simulink model "KD_cl_harness_forthao"  (R2015a)
settings: Solver=ode45  StartTime=0  StopTime=50  FixedStep=0.01  MaxStep=0.005  RelTol=1e-4  AbsTol=1e-4
InitFcn:
  | load KD_const_coeffs_0624
  | load pexhat_stuff
  | load expcon
  | load thr_ff_map
values from neighbouring files (symbols this model uses):
  c_0 = 0    [expcon.mat]
  c_1 = 1    [expcon.mat]
  c_100 = 100    [expcon.mat]
  c_1000 = 1000    [expcon.mat]
  c_10000 = 10000    [expcon.mat]
  c_1000inv = 0.0010000000475    [expcon.mat]    (also in pexhat_stuff.mat)
  c_100inv = 0.00999999977648    [expcon.mat]
  c_1_int = 1    [expcon.mat]
  c_1d2p4 = 0.416666656733    [expcon.mat]
  c_1p7 = 1.70000004768    [expcon.mat]
  c_4400inv = 0.000227272728807    [pexhat_stuff.mat]
  c_5500inv = 0.000181818177225    [expcon.mat]
  c_80 = 80    [expcon.mat]
  c_90 = 90    [expcon.mat]
  c_cal_phi = 7.6395999713e-06    [expcon.mat]
  c_compmap = [28125.0058594 29577.4082031 31350.1035156 33776.21875 37051.9296875 41026.2695312 45453.9960938 50160.3515625 55029.671875 59986.109375 64980.4296875 69980.4375 ... (320 elements, 20x16)]    [expcon.mat]
  c_ctok = 273.149993896    [expcon.mat]
  c_fflow_max = inf    [expcon.mat]
  c_fflow_min = 0    [expcon.mat]
  c_filt = 0.949999988079    [expcon.mat]
  c_flowdiv = 9.99999974738e-05    [expcon.mat]
  c_flowmin = 0    [expcon.mat]
  c_flowmult = 10000    [expcon.mat]
  c_inf = inf    [expcon.mat]
  c_km1d2k = 0.142857149243    [expcon.mat]
  c_mm3tokgpers = 2.77333338516e-08    [expcon.mat]
  c_n1 = -1    [expcon.mat]
  c_p00001 = 9.99999974738e-06    [expcon.mat]
  c_p01 = 0.00999999977648    [pexhat_stuff.mat]
  c_p016 = 0.01600000076    [expcon.mat]
  c_p1429 = 0.142900004983    [expcon.mat]
  c_p1e9 = 9.99999971718e-10    [expcon.mat]
  c_p4167 = 0.416700005531    [expcon.mat]    (also in pexhat_stuff.mat = 0.416666656733)
  c_p4d1p4 = 0.285714298487    [expcon.mat]
  c_p5401 = 0.540099978447    [expcon.mat]
  c_p9 = 0.899999976158    [expcon.mat]
  c_pincomp = 97.4216003418    [expcon.mat]
  c_ra = 287.002807617    [expcon.mat]
  c_rair = 287.09979248    [expcon.mat]
  c_Rby1000 = 0.000287000002572    [expcon.mat]
  c_roacorr = 8.05689978733e-06    [expcon.mat]
  c_rpmtoradpers = 0.104719758034    [expcon.mat]
  c_svrthrottle1 = [0.924875080585 0.575991511345 0.0858279466629 0.820202827454 0.445821881294 0.509882986546 0.0428557097912 0.753634572029 0]    [expcon.mat]
  c_svrthrottle2 = [0.145454958081 0.14545533061 0.363636374474 0.509091556072 0.509090721607 0.509091317654 0.545454084873 0.618182241917 0.145454272628]    [expcon.mat]
  c_svrthrottlearg = 0.10000000149    [expcon.mat]
  c_svrthrottlebeta = [2282.12670898 -3239.46044922 -142.784469604 -2660.34570312 1434.34350586 4150.43994141 -1580.68164062 -1039.89575195 791.34588623]    [expcon.mat]
  c_ta_max = inf    [expcon.mat]
  c_ta_min = 270    [expcon.mat]
  c_V = 0.0077999997884    [expcon.mat]
  c_vnliftmax = 90    [expcon.mat]
  c_vnliftmin = 40    [expcon.mat]
  Coefs =     [KD_const_coeffs_0624.mat]    (also in pexhat_stuff.mat)
  const =     [KD_const_coeffs_0624.mat]    (also in pexhat_stuff.mat)
  const_exhat =     [pexhat_stuff.mat]
  eegr_map =     [expcon.mat]
  egrr_delay_init = 0    [expcon.mat]
  epim_map =     [expcon.mat]
  eplufin_ff_map =     [expcon.mat]
  expcon =     [expcon.mat]
  invta = [5 5 5 5 2.5 0 0 0 0 0 0 0 ... (240 elements, 16x15)]    [expcon.mat]
  invtacols = [1000 1200 1400 1600 1800 2000 2200 2400 2600 2800 3000 3200 ... (16 elements, 1x16)]    [expcon.mat]
  IV =     [KD_const_coeffs_0624.mat]    (also in pexhat_stuff.mat)
  Lobs_init = [0 0 0]    [expcon.mat]
  map_delay_init = 120    [expcon.mat]
  maxA_t = [51.4567184448 53.8593139648 56.3063011169 58.7576789856 61.1701469421 63.4982337952 65.6955718994 67.7161483765 69.5156555176 71.0527648926 72.2902603149 73.1961746216 ... (16 elements, 1x16)]    [expcon.mat]
  obsA = [0.985195398331  0  0; -0.188821405172  1  0; 0.000342977960827  0  1]    [expcon.mat]
  sample_time = 0.016    [expcon.mat]    (also in pexhat_stuff.mat)
  SVR_EGR =     [KD_const_coeffs_0624.mat]    (also in pexhat_stuff.mat)
  SVR_EGR_exhat =     [pexhat_stuff.mat]
  SVR_throttle =     [KD_const_coeffs_0624.mat]    (also in pexhat_stuff.mat)
  uz_init = [0 0]    [expcon.mat]
undefined symbols (not defined in the file or in its folder): k1_table, k2_table, maxL, minL, Newton, Raphson
libraries: simulink x5
(part 4 of 6)

== system KD_cl_harness_forthao/ctrl_rb_explicit_20131031_v2/PID/If_Action_Subsystem1 ==
  pin : Inport
  pex : Inport  Port=2
  k : Inport  Port=3
  Action Port : ActionPort  ActionType=else
  Product10 : Product  Inputs=**  RndMeth=Zero
  Product7 : Product  Inputs=*/  RndMeth=Zero
  Product8 : Product  Inputs=**  RndMeth=Zero
  Product9 : Product  Inputs=*//  RndMeth=Zero
  Saturation : Saturate  UpperLimit=inf  LowerLimit=0
      settings: AttributesFormatString=%<LowerLimit>\n%<UpperLimit>
  Saturation2 : Saturate  UpperLimit=c_inf  LowerLimit=c_p1e9
      settings: AttributesFormatString=%<LowerLimit>\n%<UpperLimit>
  Saturation4 : Saturate  UpperLimit=c_inf  LowerLimit=c_p1e9
      settings: AttributesFormatString=%<LowerLimit>\n%<UpperLimit>
  Sqrt1 : Sqrt  AlgorithmType=Newton-Raphson  SaturateOnIntegerOverflow=on
  Sum6 : Sum  Inputs=|+-
  Sum7 : Sum  Inputs=|+-
  Sum8 : Sum  Inputs=|++
  Sum9 : Sum  Inputs=|+-
  one3 : Constant  OutDataTypeStr=single  SampleTime=sample_time
      settings: AttributesFormatString=%<Value>\n%<SampleTime>
  one4 : Constant  OutDataTypeStr=single  SampleTime=sample_time
      settings: AttributesFormatString=%<Value>\n%<SampleTime>
  one5 : Constant  OutDataTypeStr=single  SampleTime=sample_time
      settings: AttributesFormatString=%<Value>\n%<SampleTime>
  two : Constant  Value=2  OutDataTypeStr=single  SampleTime=sample_time
      settings: AttributesFormatString=%<Value>\n%<SampleTime>
  Out : Outport
  wires:
  Saturation4/1 -> Product7/2
  Saturation2/1 -> Product9/3
  Saturation/1 -> Sqrt1/1
  Sqrt1/1 -> Out/1
  Product10/1 -> Saturation/1
  Sum8/1 -> Product10/1
  [pr] -> Sum9/2
  Sum9/1 -> Product10/2
  one5/1 -> Sum9/1
  [pr] -> Sum8/2
  Product9/1 -> Sum8/1
  [pr] -> Sum6/2
  Product7/1 -> [pr]
  [k] -> Saturation2/1
  two/1 -> Product9/2
  Product8/1 -> Product9/1
  Sum7/1 -> Product8/1
  Sum6/1 -> Product8/2
  one4/1 -> Sum7/2
  [k] -> Sum7/1
  [pex] -> Saturation4/1
  [pin] -> Product7/1
  one3/1 -> Sum6/1
  pin/1 -> [pin]
  k/1 -> [k]
  pex/1 -> [pex]

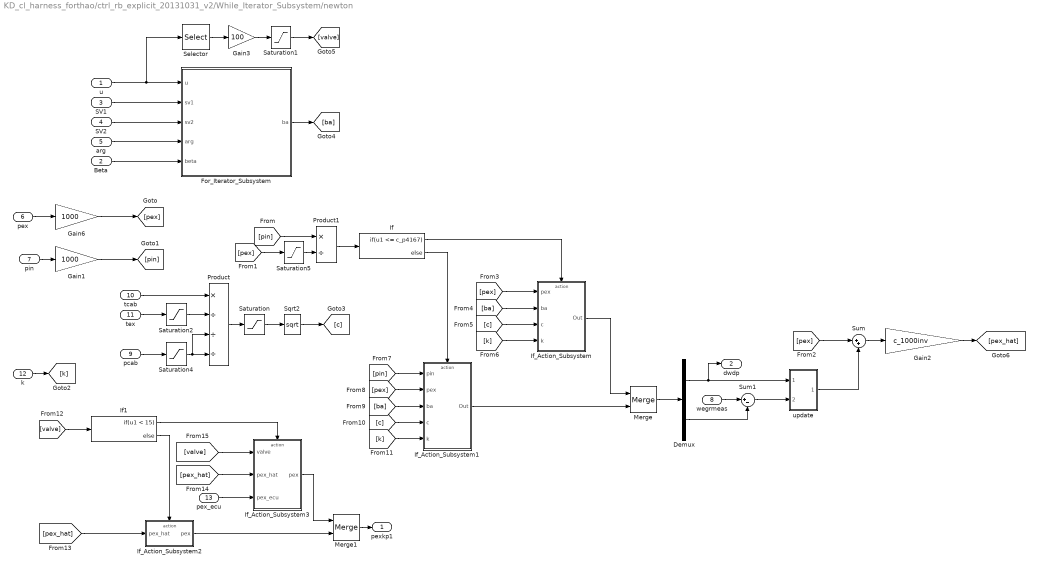
== system KD_cl_harness_forthao/ctrl_rb_explicit_20131031_v2/While_Iterator_Subsystem/newton ==
  u : Inport
  Beta : Inport  Port=2
  SV1 : Inport  Port=3
  SV2 : Inport  Port=4
  arg : Inport  Port=5
  pex : Inport  Port=6
  pin : Inport  Port=7
  wegrmeas : Inport  Port=8
  pcab : Inport  Port=9
  tcab : Inport  Port=10
  tex : Inport  Port=11
  k : Inport  Port=12
  pex_ecu : Inport  Port=13
  Demux : Demux  Outputs=2
  For_Iterator_Subsystem : Subsystem  TreatAsAtomicUnit=on
  Gain1 : Gain  Gain=1000
      settings: AttributesFormatString=%<Gain>
  Gain2 : Gain  Gain=c_1000inv
      settings: AttributesFormatString=%<Gain>
  Gain3 : Gain  Gain=100
      settings: AttributesFormatString=%<Gain>
  Gain6 : Gain  Gain=1000
      settings: AttributesFormatString=%<Gain>
  If : If  IfExpression=u1 <= c_p4167
  If1 : If  IfExpression=u1 < 15
  If_Action_Subsystem : Subsystem  TreatAsAtomicUnit=on
  If_Action_Subsystem1 : Subsystem  TreatAsAtomicUnit=on
  If_Action_Subsystem2 : Subsystem  TreatAsAtomicUnit=on
  If_Action_Subsystem3 : Subsystem  TreatAsAtomicUnit=on
  Merge : Merge
  Merge1 : Merge
  Product : Product  Inputs=*///  RndMeth=Zero
  Product1 : Product  Inputs=*/  RndMeth=Zero
  Saturation : Saturate  UpperLimit=inf  LowerLimit=0
      settings: AttributesFormatString=%<LowerLimit>\n%<UpperLimit>
  Saturation1 : Saturate  UpperLimit=c_inf  LowerLimit=c_0
      settings: AttributesFormatString=%<LowerLimit>\n%<UpperLimit>
  Saturation2 : Saturate  UpperLimit=c_inf  LowerLimit=c_p1e9
      settings: AttributesFormatString=%<LowerLimit>\n%<UpperLimit>
  Saturation4 : Saturate  UpperLimit=c_inf  LowerLimit=c_p1e9
      settings: AttributesFormatString=%<LowerLimit>\n%<UpperLimit>
  Saturation5 : Saturate  UpperLimit=c_inf  LowerLimit=c_p1e9
      settings: AttributesFormatString=%<LowerLimit>\n%<UpperLimit>
  Selector : Selector  InputPortWidth=2
  Sqrt2 : Sqrt  AlgorithmType=Newton-Raphson  SaturateOnIntegerOverflow=on
  Sum : Sum  Inputs=|++
  Sum1 : Sum  Inputs=|+-
  update : Subsystem
  pexkp1 : Outport
  dwdp : Outport  Port=2
  wires:
  Saturation5/1 -> Product1/2
  Saturation4/1 -> Product/4, Product/3
  Saturation2/1 -> Product/2
  Saturation/1 -> Sqrt2/1
  Sum/1 -> Gain2/1
  update/1(delta) -> Sum/2
  [pex] -> Sum/1
  Merge/1 -> Demux/1
  If_Action_Subsystem1/1(Out) -> Merge/2
  If_Action_Subsystem/1(Out) -> Merge/1
  [k] -> If_Action_Subsystem1/5(k)
  [c] -> If_Action_Subsystem1/4(c)
  [ba] -> If_Action_Subsystem1/3(ba)
  [pex] -> If_Action_Subsystem1/2(pex)
  [pin] -> If_Action_Subsystem1/1(pin)
  If/2 -> If_Action_Subsystem1/Action
  [k] -> If_Action_Subsystem/4(k)
  [c] -> If_Action_Subsystem/3(c)
  [ba] -> If_Action_Subsystem/2(ba)
  [pex] -> If_Action_Subsystem/1(pex)
  If/1 -> If_Action_Subsystem/Action
  Product1/1 -> If/1
  [pex] -> Saturation5/1
  [pin] -> Product1/1
  For_Iterator_Subsystem/1(ba) -> [ba]
  Product/1 -> Saturation/1
  Gain1/1 -> [pin]
  Gain6/1 -> [pex]
  SV2/1 -> For_Iterator_Subsystem/3(sv2)
  k/1 -> [k]
  tex/1 -> Saturation2/1
  tcab/1 -> Product/1
  pcab/1 -> Saturation4/1
  wegrmeas/1 -> Sum1/1
  pin/1 -> Gain1/1
  pex/1 -> Gain6/1
  arg/1 -> For_Iterator_Subsystem/4(arg)
  SV1/1 -> For_Iterator_Subsystem/2(sv1)
  Beta/1 -> For_Iterator_Subsystem/5(beta)
  u/1 -> For_Iterator_Subsystem/1(u), Selector/1
  Demux/1 -> dwdp/1, update/1(dwdp)
  Demux/2 -> Sum1/2
  Sqrt2/1 -> [c]
  Selector/1 -> Gain3/1
  Gain3/1 -> Saturation1/1
  Saturation1/1 -> [valve]
  [valve] -> If1/1
  If1/2 -> If_Action_Subsystem2/Action
  If1/1 -> If_Action_Subsystem3/Action
  Gain2/1 -> [pex_hat]
  [pex_hat] -> If_Action_Subsystem2/1(pex_hat)
  [valve] -> If_Action_Subsystem3/1(valve)
  [pex_hat] -> If_Action_Subsystem3/2(pex_hat)
  pex_ecu/1 -> If_Action_Subsystem3/3(pex_ecu)
  If_Action_Subsystem2/1(pex) -> Merge1/2
  If_Action_Subsystem3/1(pex) -> Merge1/1
  Merge1/1 -> pexkp1/1
  Sum1/1 -> update/2(error)

== system KD_cl_harness_forthao/ctrl_rb_explicit_20131031_v2/egr_est/custom_filter ==
  Input : Inport
  Data Store Read1 : DataStoreRead  DataStoreName=man_tuneFiltalpha  SampleTime=sample_time
  Data Store Read8 : DataStoreRead  DataStoreName=man_tuneFiltalpha  SampleTime=sample_time
  Delay1 : Delay  DelayLength=1  InitialCondition=0
  Product1 : Product  Inputs=**  RndMeth=Zero
  Product2 : Product  Inputs=**  RndMeth=Zero
  Saturation1 : Saturate  UpperLimit=1  LowerLimit=0
      settings: AttributesFormatString=%<LowerLimit>\n%<UpperLimit>
  Saturation4 : Saturate  UpperLimit=1  LowerLimit=0
      settings: AttributesFormatString=%<LowerLimit>\n%<UpperLimit>
  Sum1 : Sum  Inputs=+-|
  Sum11 : Sum  Inputs=++|
  man_tuneFiltalpha : Gain
  man_tuneFiltalpha1 : Gain
  zero1 : Constant  OutDataTypeStr=single  SampleTime=sample_time
      settings: AttributesFormatString=%<Value>\n%<SampleTime>
  Output : Outport  OutDataTypeStr=single
  wires:
  Input/1 -> Product1/2
  Delay1/1 -> Product2/1
  Data Store Read8/1 -> man_tuneFiltalpha1/1
  Product2/1 -> Sum11/1
  Sum1/1 -> Product1/1
  Data Store Read1/1 -> man_tuneFiltalpha/1
  Saturation4/1 -> Sum1/2
  Saturation1/1 -> Product2/2
  Product1/1 -> Sum11/2
  zero1/1 -> Sum1/1
  Sum11/1 -> Output/1, Delay1/1
  man_tuneFiltalpha/1 -> Saturation4/1
  man_tuneFiltalpha1/1 -> Saturation1/1

== system KD_cl_harness_forthao/ctrl_rb_explicit_20131031_v2/egr_est/interp ==
  valve : Inport
  MAF : Inport  Port=2
  Wcyl : Inport  Port=3
  Product : Product  RndMeth=Zero
  Product1 : Product  RndMeth=Zero
  Sum : Sum  Inputs=-+|
  Sum1 : Sum  Inputs=++|
  interp : Lookup  InputValues=[0 15]  Table=[0 1]  LookUpMeth=Interpolation-Use End Values
      settings: AttributesFormatString=%<LookUpMeth>\n%<InputValues>
  one : Constant  OutDataTypeStr=single  SampleTime=sample_time
      settings: AttributesFormatString=%<Value>\n%<SampleTime>
  Wcylhat : Outport
  wires:
  valve/1 -> interp/1
  Wcyl/1 -> Product/1
  interp/1 -> Product/2, Sum/1
  one/1 -> Sum/2
  Sum/1 -> Product1/1
  MAF/1 -> Product1/2
  Product1/1 -> Sum1/2
  Product/1 -> Sum1/1
  Sum1/1 -> Wcylhat/1

== system KD_cl_harness_forthao/ctrl_rb_explicit_20131031_v2/expcon/find_region ==
  u : Inport
  find_region : Subsystem  TreatAsAtomicUnit=on
  region_ic : Constant  Value=c_1_int  OutDataTypeStr=int32
      settings: AttributesFormatString=%<Value>
  region : Outport
  rv : Outport  Port=2
  wires:
  find_region/2(rv) -> rv/1
  find_region/1(region) -> region/1
  region_ic/1 -> find_region/2(IC)
  u/1 -> find_region/1(u)

== system KD_cl_harness_forthao/ctrl_rb_explicit_20131031_v2/expcon/get_ctrl ==
  region : Inport
  u : Inport  Port=2
  calc_u_star : Subsystem
  u_star : Outport
  wires:
  calc_u_star/1(u_star) -> u_star/1
  u/1 -> calc_u_star/2(u)
  region/1 -> calc_u_star/1(region)

== system KD_cl_harness_forthao/ctrl_rb_explicit_20131031_v2/invert_flow/valve_inversion ==
  Ro_a : Inport
  pexhaust : Inport  Port=2
  pintake : Inport  Port=3
  uwegr : Inport  Port=4
  ne_rpm : Inport  Port=5
  Cal_phi1 : Subsystem
  Constant1 : Constant  Value=c_p4167  OutDataTypeStr=single
      settings: AttributesFormatString=%<Value>
  Constant3 : Constant  Value=c_p1429  OutDataTypeStr=single
      settings: AttributesFormatString=%<Value>
  Constant4 : Constant  Value=c_1  OutDataTypeStr=single
      settings: AttributesFormatString=%<Value>
  Constant5 : Constant  Value=c_p5401  OutDataTypeStr=single
      settings: AttributesFormatString=%<Value>
  Pm_by_Pex : Product  Inputs=*/  SaturateOnIntegerOverflow=on  RndMeth=Zero  InputSameDT=on  OutDataTypeStr=Inherit: Same as first input
  Relational Operator : RelationalOperator  Operator=>  OutDataTypeStr=boolean
      settings: AttributesFormatString=%<Operator>
  Saturation1 : Saturate  UpperLimit=c_1  LowerLimit=c_p4167
      settings: AttributesFormatString=%<LowerLimit>\n%<UpperLimit>
  Saturation2 : Saturate  UpperLimit=c_inf  LowerLimit=c_90
      settings: AttributesFormatString=%<LowerLimit>\n%<UpperLimit>
  Saturation3 : Saturate  UpperLimit=c_inf  LowerLimit=c_0
      settings: AttributesFormatString=%<LowerLimit>\n%<UpperLimit>
  Saturation4 : Saturate  UpperLimit=c_inf  LowerLimit=c_p00001
      settings: AttributesFormatString=%<LowerLimit>\n%<UpperLimit>
  Sqrt : Sqrt  AlgorithmType=Newton-Raphson  SaturateOnIntegerOverflow=on
  Sum : Sum  Inputs=|+-
  Sum1 : Sum  Inputs=|++
  Switch2 : Switch  Criteria=u2 ~= 0
      settings: AttributesFormatString=%<Criteria>
  correct flow1 : Product  Inputs=*/  SaturateOnIntegerOverflow=on  RndMeth=Zero  InputSameDT=on  OutDataTypeStr=Inherit: Same as first input
  correct flow2 : Product  Inputs=**  SaturateOnIntegerOverflow=on  RndMeth=Zero  InputSameDT=on  OutDataTypeStr=Inherit: Same as first input
  correct flow3 : Product  Inputs=**  SaturateOnIntegerOverflow=on  RndMeth=Zero  InputSameDT=on  OutDataTypeStr=Inherit: Same as first input
  correct flow4 : Product  Inputs=**  SaturateOnIntegerOverflow=on  RndMeth=Zero  InputSameDT=on  OutDataTypeStr=Inherit: Same as first input
  invert_svr_lut : Lookup2D  RowIndex=invtacols  ColumnIndex=invtarows  Table=invta  LookUpMeth=Interpolation-Use End Values
      settings: AttributesFormatString=%<LookUpMeth>\n%<RowIndex>\n%<ColumnIndex>
  togps : Gain  Gain=c_1000
      settings: AttributesFormatString=%<Gain>
  valve_angle : Outport
  wires:
  Sqrt/1 -> Switch2/1
  correct flow3/1 -> Saturation3/1
  correct flow2/1 -> Sum1/1
  Constant3/1 -> correct flow2/2
  Sum/1 -> correct flow2/1, correct flow3/1
  Constant4/1 -> Sum/1
  invert_svr_lut/1 -> valve_angle/1
  uwegr/1 -> togps/1
  Ro_a/1 -> Cal_phi1/2(Ro_a)
  pexhaust/1 -> [Pex], Saturation2/1
  pintake/1 -> Pm_by_Pex/1
  Pm_by_Pex/1 -> Saturation1/1, Relational Operator/1
  Saturation1/1 -> Sum1/2, Sum/2
  [Pex] -> Cal_phi1/1(Pa)
  Sum1/1 -> correct flow3/2
  Saturation2/1 -> Pm_by_Pex/2
  Saturation3/1 -> Sqrt/1
  Saturation4/1 -> correct flow1/2
  correct flow4/1 -> Saturation4/1
  Switch2/1 -> correct flow4/2
  Cal_phi1/1(phi) -> correct flow4/1
  togps/1 -> correct flow1/1
  Relational Operator/1 -> Switch2/2
  Constant5/1 -> Switch2/3
  Constant1/1 -> Relational Operator/2
  correct flow1/1 -> invert_svr_lut/2
  ne_rpm/1 -> invert_svr_lut/1

== system KD_cl_harness_forthao/ctrl_rb_explicit_20131031_v2/ntestimator/Throttle_Model ==
  TA_deg : Inport
  Ne_rpm : Inport  Port=2
  Pim_Pa : Inport  Port=3
  Tam_K : Inport  Port=4
  wegrthr : Inport  Port=5
  Air_Model_map_use : Subsystem
  Ra : Constant  Value=c_rair  OutDataTypeStr=single  SampleTime=sample_time
      settings: AttributesFormatString=%<Value>\n%<SampleTime>
  p_pre_throttle : Outport  OutDataTypeStr=single
  wires:
  TA_deg/1 -> Air_Model_map_use/1(TA_deg)
  Tam_K/1 -> Air_Model_map_use/4(Ta_K)
  Pim_Pa/1 -> Air_Model_map_use/3(Pim_Pa)
  Ra/1 -> Air_Model_map_use/5(R_a)
  Ne_rpm/1 -> Air_Model_map_use/2(Ne_rpm)
  wegrthr/1 -> Air_Model_map_use/6(wegrthr)
  Air_Model_map_use/1(p_pre_throttle) -> p_pre_throttle/1

== system KD_cl_harness_forthao/ctrl_rb_explicit_20131031_v2/ntestimator/custom_filter ==
  Input : Inport
  Delay1 : Delay  DelayLength=1  InitialCondition=0
  Product1 : Product  Inputs=**  RndMeth=Zero
  Product2 : Product  Inputs=**  RndMeth=Zero
  Saturation1 : Saturate  UpperLimit=1  LowerLimit=0
      settings: AttributesFormatString=%<LowerLimit>\n%<UpperLimit>
  Saturation4 : Saturate  UpperLimit=1  LowerLimit=0
      settings: AttributesFormatString=%<LowerLimit>\n%<UpperLimit>
  Sum1 : Sum  Inputs=+-|
  Sum11 : Sum  Inputs=++|
  filt : Constant  Value=c_filt  OutDataTypeStr=single  SampleTime=sample_time
      settings: AttributesFormatString=%<Value>\n%<SampleTime>
  filt1 : Constant  Value=c_filt  OutDataTypeStr=single  SampleTime=sample_time
      settings: AttributesFormatString=%<Value>\n%<SampleTime>
  one : Constant  OutDataTypeStr=single  SampleTime=sample_time
      settings: AttributesFormatString=%<Value>\n%<SampleTime>
  Output : Outport  OutDataTypeStr=single
  wires:
  Input/1 -> Product1/2
  Delay1/1 -> Product2/1
  filt/1 -> Saturation1/1
  Product2/1 -> Sum11/1
  Sum1/1 -> Product1/1
  filt1/1 -> Saturation4/1
  Saturation4/1 -> Sum1/2
  Saturation1/1 -> Product2/2
  Product1/1 -> Sum11/2
  one/1 -> Sum1/1
  Sum11/1 -> Output/1, Delay1/1

== system KD_cl_harness_forthao/ctrl_rb_explicit_20131031_v2/rpm1200testpattern/IfActionSubsystem ==
  Action Port : ActionPort  ActionType=then
  tp : Constant  Value=[150;50;150]  OutDataTypeStr=single  SampleTime=sample_time
      settings: AttributesFormatString=%<Value>\n%<SampleTime>
  Out1 : Outport  InitialOutput=[150;50;150]
  wires:
  tp/1 -> Out1/1

== system KD_cl_harness_forthao/ctrl_rb_explicit_20131031_v2/rpm1200testpattern/IfActionSubsystem1 ==
  Action Port : ActionPort  ActionType=elseif
  tp : Constant  Value=[150;50;150]  OutDataTypeStr=single  SampleTime=sample_time
      settings: AttributesFormatString=%<Value>\n%<SampleTime>
  Out1 : Outport  InitialOutput=[150;50;150]
  wires:
  tp/1 -> Out1/1

== system KD_cl_harness_forthao/ctrl_rb_explicit_20131031_v2/rpm1200testpattern/IfActionSubsystem10 ==
  Action Port : ActionPort  ActionType=elseif
  tp : Constant  Value=[150;50;150]  OutDataTypeStr=single  SampleTime=sample_time
      settings: AttributesFormatString=%<Value>\n%<SampleTime>
  Out1 : Outport  InitialOutput=[150;50;150]
  wires:
  tp/1 -> Out1/1

== system KD_cl_harness_forthao/ctrl_rb_explicit_20131031_v2/rpm1200testpattern/IfActionSubsystem11 ==
  Action Port : ActionPort  ActionType=elseif
  tp : Constant  Value=[150;50;150]  OutDataTypeStr=single  SampleTime=sample_time
      settings: AttributesFormatString=%<Value>\n%<SampleTime>
  Out1 : Outport  InitialOutput=[150;50;150]
  wires:
  tp/1 -> Out1/1

== system KD_cl_harness_forthao/ctrl_rb_explicit_20131031_v2/rpm1200testpattern/IfActionSubsystem12 ==
  Action Port : ActionPort  ActionType=elseif
  tp : Constant  Value=[150;50;150]  OutDataTypeStr=single  SampleTime=sample_time
      settings: AttributesFormatString=%<Value>\n%<SampleTime>
  Out1 : Outport  InitialOutput=[150;50;150]
  wires:
  tp/1 -> Out1/1

== system KD_cl_harness_forthao/ctrl_rb_explicit_20131031_v2/rpm1200testpattern/IfActionSubsystem13 ==
  Action Port : ActionPort  ActionType=elseif
  tp : Constant  Value=[150;50;150]  OutDataTypeStr=single  SampleTime=sample_time
      settings: AttributesFormatString=%<Value>\n%<SampleTime>
  Out1 : Outport  InitialOutput=[150;50;150]
  wires:
  tp/1 -> Out1/1

== system KD_cl_harness_forthao/ctrl_rb_explicit_20131031_v2/rpm1200testpattern/IfActionSubsystem14 ==
  Action Port : ActionPort  ActionType=elseif
  tp : Constant  Value=[150;50;150]  OutDataTypeStr=single  SampleTime=sample_time
      settings: AttributesFormatString=%<Value>\n%<SampleTime>
  Out1 : Outport  InitialOutput=[150;50;150]
  wires:
  tp/1 -> Out1/1

== system KD_cl_harness_forthao/ctrl_rb_explicit_20131031_v2/rpm1200testpattern/IfActionSubsystem15 ==
  Action Port : ActionPort  ActionType=elseif
  tp : Constant  Value=[150;20;150]  OutDataTypeStr=single  SampleTime=sample_time
      settings: AttributesFormatString=%<Value>\n%<SampleTime>
  Out1 : Outport  InitialOutput=[150;20;150]
  wires:
  tp/1 -> Out1/1

== system KD_cl_harness_forthao/ctrl_rb_explicit_20131031_v2/rpm1200testpattern/IfActionSubsystem16 ==
  Action Port : ActionPort  ActionType=elseif
  tp : Constant  Value=[150;5;150]  OutDataTypeStr=single  SampleTime=sample_time
      settings: AttributesFormatString=%<Value>\n%<SampleTime>
  Out1 : Outport  InitialOutput=[150;5;150]
  wires:
  tp/1 -> Out1/1

== system KD_cl_harness_forthao/ctrl_rb_explicit_20131031_v2/rpm1200testpattern/IfActionSubsystem17 ==
  Action Port : ActionPort  ActionType=elseif
  tp : Constant  Value=[150;15;150]  OutDataTypeStr=single  SampleTime=sample_time
      settings: AttributesFormatString=%<Value>\n%<SampleTime>
  Out1 : Outport  InitialOutput=[150;15;150]
  wires:
  tp/1 -> Out1/1

== system KD_cl_harness_forthao/ctrl_rb_explicit_20131031_v2/rpm1200testpattern/IfActionSubsystem18 ==
  Action Port : ActionPort  ActionType=elseif
  tp : Constant  Value=[130;20;150]  OutDataTypeStr=single  SampleTime=sample_time
      settings: AttributesFormatString=%<Value>\n%<SampleTime>
  Out1 : Outport  InitialOutput=[130;20;150]
  wires:
  tp/1 -> Out1/1

== system KD_cl_harness_forthao/ctrl_rb_explicit_20131031_v2/rpm1200testpattern/IfActionSubsystem19 ==
  Action Port : ActionPort  ActionType=elseif
  tp : Constant  Value=[130;20;115]  OutDataTypeStr=single  SampleTime=sample_time
      settings: AttributesFormatString=%<Value>\n%<SampleTime>
  Out1 : Outport  InitialOutput=[130;20;115]
  wires:
  tp/1 -> Out1/1

== system KD_cl_harness_forthao/ctrl_rb_explicit_20131031_v2/rpm1200testpattern/IfActionSubsystem2 ==
  Action Port : ActionPort  ActionType=elseif
  tp : Constant  Value=[150;50;150]  OutDataTypeStr=single  SampleTime=sample_time
      settings: AttributesFormatString=%<Value>\n%<SampleTime>
  Out1 : Outport  InitialOutput=[150;50;150]
  wires:
  tp/1 -> Out1/1

== system KD_cl_harness_forthao/ctrl_rb_explicit_20131031_v2/rpm1200testpattern/IfActionSubsystem20 ==
  Action Port : ActionPort  ActionType=elseif
  tp : Constant  Value=[130;20;110]  OutDataTypeStr=single  SampleTime=sample_time
      settings: AttributesFormatString=%<Value>\n%<SampleTime>
  Out1 : Outport  InitialOutput=[130;20;110]
  wires:
  tp/1 -> Out1/1

== system KD_cl_harness_forthao/ctrl_rb_explicit_20131031_v2/rpm1200testpattern/IfActionSubsystem21 ==
  Action Port : ActionPort  ActionType=elseif
  tp : Constant  Value=[130;20;105]  OutDataTypeStr=single  SampleTime=sample_time
      settings: AttributesFormatString=%<Value>\n%<SampleTime>
  Out1 : Outport  InitialOutput=[130;20;105]
  wires:
  tp/1 -> Out1/1

== system KD_cl_harness_forthao/ctrl_rb_explicit_20131031_v2/rpm1200testpattern/IfActionSubsystem22 ==
  Action Port : ActionPort  ActionType=elseif
  tp : Constant  Value=[130;0;105]  OutDataTypeStr=single  SampleTime=sample_time
      settings: AttributesFormatString=%<Value>\n%<SampleTime>
  Out1 : Outport  InitialOutput=[130;0;105]
  wires:
  tp/1 -> Out1/1

== system KD_cl_harness_forthao/ctrl_rb_explicit_20131031_v2/rpm1200testpattern/IfActionSubsystem23 ==
  Action Port : ActionPort  ActionType=elseif
  tp : Constant  Value=[130;0;110]  OutDataTypeStr=single  SampleTime=sample_time
      settings: AttributesFormatString=%<Value>\n%<SampleTime>
  Out1 : Outport  InitialOutput=[130;0;110]
  wires:
  tp/1 -> Out1/1

== system KD_cl_harness_forthao/ctrl_rb_explicit_20131031_v2/rpm1200testpattern/IfActionSubsystem24 ==
  Action Port : ActionPort  ActionType=elseif
  tp : Constant  Value=[150;3;150]  OutDataTypeStr=single  SampleTime=sample_time
      settings: AttributesFormatString=%<Value>\n%<SampleTime>
  Out1 : Outport  InitialOutput=[150;3;150]
  wires:
  tp/1 -> Out1/1

== system KD_cl_harness_forthao/ctrl_rb_explicit_20131031_v2/rpm1200testpattern/IfActionSubsystem25 ==
  Action Port : ActionPort  ActionType=elseif
  tp : Constant  Value=[150;10;150]  OutDataTypeStr=single  SampleTime=sample_time
      settings: AttributesFormatString=%<Value>\n%<SampleTime>
  Out1 : Outport  InitialOutput=[150;10;150]
  wires:
  tp/1 -> Out1/1

== system KD_cl_harness_forthao/ctrl_rb_explicit_20131031_v2/rpm1200testpattern/IfActionSubsystem26 ==
  Action Port : ActionPort  ActionType=elseif
  tp : Constant  Value=[150;20;150]  OutDataTypeStr=single  SampleTime=sample_time
      settings: AttributesFormatString=%<Value>\n%<SampleTime>
  Out1 : Outport  InitialOutput=[150;20;150]
  wires:
  tp/1 -> Out1/1

== system KD_cl_harness_forthao/ctrl_rb_explicit_20131031_v2/rpm1200testpattern/IfActionSubsystem27 ==
  Action Port : ActionPort  ActionType=elseif
  tp : Constant  Value=[150;20;150]  OutDataTypeStr=single  SampleTime=sample_time
      settings: AttributesFormatString=%<Value>\n%<SampleTime>
  Out1 : Outport  InitialOutput=[150;20;150]
  wires:
  tp/1 -> Out1/1

== system KD_cl_harness_forthao/ctrl_rb_explicit_20131031_v2/rpm1200testpattern/IfActionSubsystem28 ==
  Action Port : ActionPort  ActionType=elseif
  tp : Constant  Value=[110;20;150]  OutDataTypeStr=single  SampleTime=sample_time
      settings: AttributesFormatString=%<Value>\n%<SampleTime>
  Out1 : Outport  InitialOutput=[110;20;150]
  wires:
  tp/1 -> Out1/1

== system KD_cl_harness_forthao/ctrl_rb_explicit_20131031_v2/rpm1200testpattern/IfActionSubsystem29 ==
  Action Port : ActionPort  ActionType=elseif
  tp : Constant  Value=[100;20;150]  OutDataTypeStr=single  SampleTime=sample_time
      settings: AttributesFormatString=%<Value>\n%<SampleTime>
  Out1 : Outport  InitialOutput=[100;20;150]
  wires:
  tp/1 -> Out1/1

== system KD_cl_harness_forthao/ctrl_rb_explicit_20131031_v2/rpm1200testpattern/IfActionSubsystem3 ==
  Action Port : ActionPort  ActionType=elseif
  tp : Constant  Value=[150;50;150]  OutDataTypeStr=single  SampleTime=sample_time
      settings: AttributesFormatString=%<Value>\n%<SampleTime>
  Out1 : Outport  InitialOutput=[150;50;150]
  wires:
  tp/1 -> Out1/1

== system KD_cl_harness_forthao/ctrl_rb_explicit_20131031_v2/rpm1200testpattern/IfActionSubsystem30 ==
  Action Port : ActionPort  ActionType=elseif
  tp : Constant  Value=[115;20;150]  OutDataTypeStr=single  SampleTime=sample_time
      settings: AttributesFormatString=%<Value>\n%<SampleTime>
  Out1 : Outport  InitialOutput=[115;20;150]
  wires:
  tp/1 -> Out1/1

== system KD_cl_harness_forthao/ctrl_rb_explicit_20131031_v2/rpm1200testpattern/IfActionSubsystem31 ==
  Action Port : ActionPort  ActionType=elseif
  tp : Constant  Value=[105;20;150]  OutDataTypeStr=single  SampleTime=sample_time
      settings: AttributesFormatString=%<Value>\n%<SampleTime>
  Out1 : Outport  InitialOutput=[105;20;150]
  wires:
  tp/1 -> Out1/1

== system KD_cl_harness_forthao/ctrl_rb_explicit_20131031_v2/rpm1200testpattern/IfActionSubsystem32 ==
  Action Port : ActionPort  ActionType=elseif
  tp : Constant  Value=[105;0;110]  OutDataTypeStr=single  SampleTime=sample_time
      settings: AttributesFormatString=%<Value>\n%<SampleTime>
  Out1 : Outport  InitialOutput=[105;0;110]
  wires:
  tp/1 -> Out1/1

== system KD_cl_harness_forthao/ctrl_rb_explicit_20131031_v2/rpm1200testpattern/IfActionSubsystem33 ==
  Action Port : ActionPort  ActionType=elseif
  tp : Constant  Value=[100;0;110]  OutDataTypeStr=single  SampleTime=sample_time
      settings: AttributesFormatString=%<Value>\n%<SampleTime>
  Out1 : Outport  InitialOutput=[100;0;110]
  wires:
  tp/1 -> Out1/1

== system KD_cl_harness_forthao/ctrl_rb_explicit_20131031_v2/rpm1200testpattern/IfActionSubsystem34 ==
  Action Port : ActionPort  ActionType=else
  tp : Constant  Value=[150;50;150]  OutDataTypeStr=single  SampleTime=sample_time
      settings: AttributesFormatString=%<Value>\n%<SampleTime>
  Out1 : Outport  InitialOutput=[150;50;150]
  wires:
  tp/1 -> Out1/1

== system KD_cl_harness_forthao/ctrl_rb_explicit_20131031_v2/rpm1200testpattern/IfActionSubsystem4 ==
  Action Port : ActionPort  ActionType=elseif
  tp : Constant  Value=[150;50;150]  OutDataTypeStr=single  SampleTime=sample_time
      settings: AttributesFormatString=%<Value>\n%<SampleTime>
  Out1 : Outport  InitialOutput=[150;50;150]
  wires:
  tp/1 -> Out1/1

== system KD_cl_harness_forthao/ctrl_rb_explicit_20131031_v2/rpm1200testpattern/IfActionSubsystem5 ==
  Action Port : ActionPort  ActionType=elseif
  tp : Constant  Value=[150;50;150]  OutDataTypeStr=single  SampleTime=sample_time
      settings: AttributesFormatString=%<Value>\n%<SampleTime>
  Out1 : Outport  InitialOutput=[150;50;150]
  wires:
  tp/1 -> Out1/1

== system KD_cl_harness_forthao/ctrl_rb_explicit_20131031_v2/rpm1200testpattern/IfActionSubsystem6 ==
  Action Port : ActionPort  ActionType=elseif
  tp : Constant  Value=[150;50;150]  OutDataTypeStr=single  SampleTime=sample_time
      settings: AttributesFormatString=%<Value>\n%<SampleTime>
  Out1 : Outport  InitialOutput=[150;50;150]
  wires:
  tp/1 -> Out1/1

== system KD_cl_harness_forthao/ctrl_rb_explicit_20131031_v2/rpm1200testpattern/IfActionSubsystem7 ==
  Action Port : ActionPort  ActionType=elseif
  tp : Constant  Value=[150;50;150]  OutDataTypeStr=single  SampleTime=sample_time
      settings: AttributesFormatString=%<Value>\n%<SampleTime>
  Out1 : Outport  InitialOutput=[150;50;150]
  wires:
  tp/1 -> Out1/1

== system KD_cl_harness_forthao/ctrl_rb_explicit_20131031_v2/rpm1200testpattern/IfActionSubsystem8 ==
  Action Port : ActionPort  ActionType=elseif
  tp : Constant  Value=[150;50;150]  OutDataTypeStr=single  SampleTime=sample_time
      settings: AttributesFormatString=%<Value>\n%<SampleTime>
  Out1 : Outport  InitialOutput=[150;50;150]
  wires:
  tp/1 -> Out1/1

== system KD_cl_harness_forthao/ctrl_rb_explicit_20131031_v2/rpm1200testpattern/IfActionSubsystem9 ==
  Action Port : ActionPort  ActionType=elseif
  tp : Constant  Value=[150;50;150]  OutDataTypeStr=single  SampleTime=sample_time
      settings: AttributesFormatString=%<Value>\n%<SampleTime>
  Out1 : Outport  InitialOutput=[150;50;150]
  wires:
  tp/1 -> Out1/1

== system KD_cl_harness_forthao/ctrl_rb_explicit_20131031_v2/rpm2500testpattern/IfActionSubsystem ==
  Action Port : ActionPort  ActionType=then
  tp : Constant  Value=[170;50;250]  OutDataTypeStr=single  SampleTime=sample_time
      settings: AttributesFormatString=%<Value>\n%<SampleTime>
  Out1 : Outport  InitialOutput=[170;50;250]
  wires:
  tp/1 -> Out1/1

== system KD_cl_harness_forthao/ctrl_rb_explicit_20131031_v2/rpm2500testpattern/IfActionSubsystem1 ==
  Action Port : ActionPort  ActionType=elseif
  tp : Constant  Value=[170;50;250]  OutDataTypeStr=single  SampleTime=sample_time
      settings: AttributesFormatString=%<Value>\n%<SampleTime>
  Out1 : Outport  InitialOutput=[170;50;250]
  wires:
  tp/1 -> Out1/1

== system KD_cl_harness_forthao/ctrl_rb_explicit_20131031_v2/rpm2500testpattern/IfActionSubsystem10 ==
  Action Port : ActionPort  ActionType=elseif
  tp : Constant  Value=[160;50;250]  OutDataTypeStr=single  SampleTime=sample_time
      settings: AttributesFormatString=%<Value>\n%<SampleTime>
  Out1 : Outport  InitialOutput=[160;50;250]
  wires:
  tp/1 -> Out1/1

== system KD_cl_harness_forthao/ctrl_rb_explicit_20131031_v2/rpm2500testpattern/IfActionSubsystem11 ==
  Action Port : ActionPort  ActionType=elseif
  tp : Constant  Value=[160;0;250]  OutDataTypeStr=single  SampleTime=sample_time
      settings: AttributesFormatString=%<Value>\n%<SampleTime>
  Out1 : Outport  InitialOutput=[160;0;250]
  wires:
  tp/1 -> Out1/1

== system KD_cl_harness_forthao/ctrl_rb_explicit_20131031_v2/rpm2500testpattern/IfActionSubsystem12 ==
  Action Port : ActionPort  ActionType=elseif
  tp : Constant  Value=[160;15;250]  OutDataTypeStr=single  SampleTime=sample_time
      settings: AttributesFormatString=%<Value>\n%<SampleTime>
  Out1 : Outport  InitialOutput=[160;15;250]
  wires:
  tp/1 -> Out1/1

== system KD_cl_harness_forthao/ctrl_rb_explicit_20131031_v2/rpm2500testpattern/IfActionSubsystem13 ==
  Action Port : ActionPort  ActionType=elseif
  tp : Constant  Value=[160;3;250]  OutDataTypeStr=single  SampleTime=sample_time
      settings: AttributesFormatString=%<Value>\n%<SampleTime>
  Out1 : Outport  InitialOutput=[160;3;250]
  wires:
  tp/1 -> Out1/1

== system KD_cl_harness_forthao/ctrl_rb_explicit_20131031_v2/rpm2500testpattern/IfActionSubsystem14 ==
  Action Port : ActionPort  ActionType=elseif
  tp : Constant  Value=[150;3;250]  OutDataTypeStr=single  SampleTime=sample_time
      settings: AttributesFormatString=%<Value>\n%<SampleTime>
  Out1 : Outport  InitialOutput=[150;3;250]
  wires:
  tp/1 -> Out1/1

== system KD_cl_harness_forthao/ctrl_rb_explicit_20131031_v2/rpm2500testpattern/IfActionSubsystem15 ==
  Action Port : ActionPort  ActionType=elseif
  tp : Constant  Value=[140;3;250]  OutDataTypeStr=single  SampleTime=sample_time
      settings: AttributesFormatString=%<Value>\n%<SampleTime>
  Out1 : Outport  InitialOutput=[140;3;250]
  wires:
  tp/1 -> Out1/1

== system KD_cl_harness_forthao/ctrl_rb_explicit_20131031_v2/rpm2500testpattern/IfActionSubsystem16 ==
  Action Port : ActionPort  ActionType=elseif
  tp : Constant  Value=[140;0;250]  OutDataTypeStr=single  SampleTime=sample_time
      settings: AttributesFormatString=%<Value>\n%<SampleTime>
  Out1 : Outport  InitialOutput=[140;0;250]
  wires:
  tp/1 -> Out1/1

== system KD_cl_harness_forthao/ctrl_rb_explicit_20131031_v2/rpm2500testpattern/IfActionSubsystem17 ==
  Action Port : ActionPort  ActionType=elseif
  tp : Constant  Value=[140;20;250]  OutDataTypeStr=single  SampleTime=sample_time
      settings: AttributesFormatString=%<Value>\n%<SampleTime>
  Out1 : Outport  InitialOutput=[140;20;250]
  wires:
  tp/1 -> Out1/1

== system KD_cl_harness_forthao/ctrl_rb_explicit_20131031_v2/rpm2500testpattern/IfActionSubsystem18 ==
  Action Port : ActionPort  ActionType=elseif
  tp : Constant  Value=[140;0;110]  OutDataTypeStr=single  SampleTime=sample_time
      settings: AttributesFormatString=%<Value>\n%<SampleTime>
  Out1 : Outport  InitialOutput=[140;0;110]
  wires:
  tp/1 -> Out1/1

== system KD_cl_harness_forthao/ctrl_rb_explicit_20131031_v2/rpm2500testpattern/IfActionSubsystem19 ==
  Action Port : ActionPort  ActionType=elseif
  tp : Constant  Value=[140;10;110]  OutDataTypeStr=single  SampleTime=sample_time
      settings: AttributesFormatString=%<Value>\n%<SampleTime>
  Out1 : Outport  InitialOutput=[140;10;110]
  wires:
  tp/1 -> Out1/1

== system KD_cl_harness_forthao/ctrl_rb_explicit_20131031_v2/rpm2500testpattern/IfActionSubsystem2 ==
  Action Port : ActionPort  ActionType=elseif
  tp : Constant  Value=[170;50;250]  OutDataTypeStr=single  SampleTime=sample_time
      settings: AttributesFormatString=%<Value>\n%<SampleTime>
  Out1 : Outport  InitialOutput=[170;50;250]
  wires:
  tp/1 -> Out1/1

== system KD_cl_harness_forthao/ctrl_rb_explicit_20131031_v2/rpm2500testpattern/IfActionSubsystem20 ==
  Action Port : ActionPort  ActionType=elseif
  tp : Constant  Value=[140;10;120]  OutDataTypeStr=single  SampleTime=sample_time
      settings: AttributesFormatString=%<Value>\n%<SampleTime>
  Out1 : Outport  InitialOutput=[140;10;120]
  wires:
  tp/1 -> Out1/1

== system KD_cl_harness_forthao/ctrl_rb_explicit_20131031_v2/rpm2500testpattern/IfActionSubsystem21 ==
  Action Port : ActionPort  ActionType=elseif
  tp : Constant  Value=[140;10;150]  OutDataTypeStr=single  SampleTime=sample_time
      settings: AttributesFormatString=%<Value>\n%<SampleTime>
  Out1 : Outport  InitialOutput=[140;10;150]
  wires:
  tp/1 -> Out1/1

== system KD_cl_harness_forthao/ctrl_rb_explicit_20131031_v2/rpm2500testpattern/IfActionSubsystem22 ==
  Action Port : ActionPort  ActionType=elseif
  tp : Constant  Value=[140;10;110]  OutDataTypeStr=single  SampleTime=sample_time
      settings: AttributesFormatString=%<Value>\n%<SampleTime>
  Out1 : Outport  InitialOutput=[140;10;110]
  wires:
  tp/1 -> Out1/1

== system KD_cl_harness_forthao/ctrl_rb_explicit_20131031_v2/rpm2500testpattern/IfActionSubsystem23 ==
  Action Port : ActionPort  ActionType=elseif
  tp : Constant  Value=[140;10;150]  OutDataTypeStr=single  SampleTime=sample_time
      settings: AttributesFormatString=%<Value>\n%<SampleTime>
  Out1 : Outport  InitialOutput=[140;10;150]
  wires:
  tp/1 -> Out1/1

== system KD_cl_harness_forthao/ctrl_rb_explicit_20131031_v2/rpm2500testpattern/IfActionSubsystem24 ==
  Action Port : ActionPort  ActionType=elseif
  tp : Constant  Value=[140;20;250]  OutDataTypeStr=single  SampleTime=sample_time
      settings: AttributesFormatString=%<Value>\n%<SampleTime>
  Out1 : Outport  InitialOutput=[140;20;250]
  wires:
  tp/1 -> Out1/1

== system KD_cl_harness_forthao/ctrl_rb_explicit_20131031_v2/rpm2500testpattern/IfActionSubsystem25 ==
  Action Port : ActionPort  ActionType=elseif
  tp : Constant  Value=[140;20;250]  OutDataTypeStr=single  SampleTime=sample_time
      settings: AttributesFormatString=%<Value>\n%<SampleTime>
  Out1 : Outport  InitialOutput=[140;20;250]
  wires:
  tp/1 -> Out1/1

== system KD_cl_harness_forthao/ctrl_rb_explicit_20131031_v2/rpm2500testpattern/IfActionSubsystem26 ==
  Action Port : ActionPort  ActionType=elseif
  tp : Constant  Value=[140;20;250]  OutDataTypeStr=single  SampleTime=sample_time
      settings: AttributesFormatString=%<Value>\n%<SampleTime>
  Out1 : Outport  InitialOutput=[140;20;250]
  wires:
  tp/1 -> Out1/1

== system KD_cl_harness_forthao/ctrl_rb_explicit_20131031_v2/rpm2500testpattern/IfActionSubsystem27 ==
  Action Port : ActionPort  ActionType=elseif
  tp : Constant  Value=[140;20;250]  OutDataTypeStr=single  SampleTime=sample_time
      settings: AttributesFormatString=%<Value>\n%<SampleTime>
  Out1 : Outport  InitialOutput=[140;20;250]
  wires:
  tp/1 -> Out1/1

== system KD_cl_harness_forthao/ctrl_rb_explicit_20131031_v2/rpm2500testpattern/IfActionSubsystem28 ==
  Action Port : ActionPort  ActionType=elseif
  tp : Constant  Value=[140;20;250]  OutDataTypeStr=single  SampleTime=sample_time
      settings: AttributesFormatString=%<Value>\n%<SampleTime>
  Out1 : Outport  InitialOutput=[140;20;250]
  wires:
  tp/1 -> Out1/1

== system KD_cl_harness_forthao/ctrl_rb_explicit_20131031_v2/rpm2500testpattern/IfActionSubsystem29 ==
  Action Port : ActionPort  ActionType=elseif
  tp : Constant  Value=[140;20;125]  OutDataTypeStr=single  SampleTime=sample_time
      settings: AttributesFormatString=%<Value>\n%<SampleTime>
  Out1 : Outport  InitialOutput=[140;20;125]
  wires:
  tp/1 -> Out1/1

== system KD_cl_harness_forthao/ctrl_rb_explicit_20131031_v2/rpm2500testpattern/IfActionSubsystem3 ==
  Action Port : ActionPort  ActionType=elseif
  tp : Constant  Value=[158;50;250]  OutDataTypeStr=single  SampleTime=sample_time
      settings: AttributesFormatString=%<Value>\n%<SampleTime>
  Out1 : Outport  InitialOutput=[158;50;250]
  wires:
  tp/1 -> Out1/1

== system KD_cl_harness_forthao/ctrl_rb_explicit_20131031_v2/rpm2500testpattern/IfActionSubsystem30 ==
  Action Port : ActionPort  ActionType=elseif
  tp : Constant  Value=[140;20;120]  OutDataTypeStr=single  SampleTime=sample_time
      settings: AttributesFormatString=%<Value>\n%<SampleTime>
  Out1 : Outport  InitialOutput=[140;20;120]
  wires:
  tp/1 -> Out1/1

== system KD_cl_harness_forthao/ctrl_rb_explicit_20131031_v2/rpm2500testpattern/IfActionSubsystem31 ==
  Action Port : ActionPort  ActionType=elseif
  tp : Constant  Value=[140;20;110]  OutDataTypeStr=single  SampleTime=sample_time
      settings: AttributesFormatString=%<Value>\n%<SampleTime>
  Out1 : Outport  InitialOutput=[140;20;110]
  wires:
  tp/1 -> Out1/1

== system KD_cl_harness_forthao/ctrl_rb_explicit_20131031_v2/rpm2500testpattern/IfActionSubsystem32 ==
  Action Port : ActionPort  ActionType=else
  tp : Constant  Value=[170;50;250]  OutDataTypeStr=single  SampleTime=sample_time
      settings: AttributesFormatString=%<Value>\n%<SampleTime>
  Out1 : Outport  InitialOutput=[170;50;250]
  wires:
  tp/1 -> Out1/1

== system KD_cl_harness_forthao/ctrl_rb_explicit_20131031_v2/rpm2500testpattern/IfActionSubsystem4 ==
  Action Port : ActionPort  ActionType=elseif
  tp : Constant  Value=[158;50;250]  OutDataTypeStr=single  SampleTime=sample_time
      settings: AttributesFormatString=%<Value>\n%<SampleTime>
  Out1 : Outport  InitialOutput=[158;50;250]
  wires:
  tp/1 -> Out1/1

== system KD_cl_harness_forthao/ctrl_rb_explicit_20131031_v2/rpm2500testpattern/IfActionSubsystem5 ==
  Action Port : ActionPort  ActionType=elseif
  tp : Constant  Value=[158;50;250]  OutDataTypeStr=single  SampleTime=sample_time
      settings: AttributesFormatString=%<Value>\n%<SampleTime>
  Out1 : Outport  InitialOutput=[158;50;250]
  wires:
  tp/1 -> Out1/1

== system KD_cl_harness_forthao/ctrl_rb_explicit_20131031_v2/rpm2500testpattern/IfActionSubsystem6 ==
  Action Port : ActionPort  ActionType=elseif
  tp : Constant  Value=[158;50;250]  OutDataTypeStr=single  SampleTime=sample_time
      settings: AttributesFormatString=%<Value>\n%<SampleTime>
  Out1 : Outport  InitialOutput=[158;50;250]
  wires:
  tp/1 -> Out1/1

== system KD_cl_harness_forthao/ctrl_rb_explicit_20131031_v2/rpm2500testpattern/IfActionSubsystem7 ==
  Action Port : ActionPort  ActionType=elseif
  tp : Constant  Value=[150;50;250]  OutDataTypeStr=single  SampleTime=sample_time
      settings: AttributesFormatString=%<Value>\n%<SampleTime>
  Out1 : Outport  InitialOutput=[150;50;250]
  wires:
  tp/1 -> Out1/1

== system KD_cl_harness_forthao/ctrl_rb_explicit_20131031_v2/rpm2500testpattern/IfActionSubsystem8 ==
  Action Port : ActionPort  ActionType=elseif
  tp : Constant  Value=[170;50;250]  OutDataTypeStr=single  SampleTime=sample_time
      settings: AttributesFormatString=%<Value>\n%<SampleTime>
  Out1 : Outport  InitialOutput=[170;50;250]
  wires:
  tp/1 -> Out1/1

== system KD_cl_harness_forthao/ctrl_rb_explicit_20131031_v2/rpm2500testpattern/IfActionSubsystem9 ==
  Action Port : ActionPort  ActionType=elseif
  tp : Constant  Value=[140;50;250]  OutDataTypeStr=single  SampleTime=sample_time
      settings: AttributesFormatString=%<Value>\n%<SampleTime>
  Out1 : Outport  InitialOutput=[140;50;250]
  wires:
  tp/1 -> Out1/1

== system KD_cl_harness_forthao/ctrl_rb_explicit_20131031_v2/set_point_maps/EGR_rate_map ==
  fuel_rate_mm3perst : Inport
  engine_speed : Inport  Port=2
  Gain2 : Gain  Gain=c_100
      settings: AttributesFormatString=%<Gain>
  epimbs_map : Lookup2D  RowIndex=eegr_map.x  ColumnIndex=eegr_map.y  Table=eegr_map.z  LookUpMeth=Interpolation-Use End Values
      settings: AttributesFormatString=%<LookUpMeth>\n%<RowIndex>\n%<ColumnIndex>
  EGR_rate_ref : Outport
  wires:
  epimbs_map/1 -> Gain2/1
  Gain2/1 -> EGR_rate_ref/1
  fuel_rate_mm3perst/1 -> epimbs_map/2
  engine_speed/1 -> epimbs_map/1

== system KD_cl_harness_forthao/ctrl_rb_explicit_20131031_v2/set_point_maps/intake_pressure_map ==
  fuel_rate_mm3perst : Inport
  engine_speed : Inport  Port=2
  boost_pressure_map : Subsystem
  intake_manifold_pressure_ref : Outport
  wires:
  engine_speed/1 -> boost_pressure_map/2(engine_speed)
  fuel_rate_mm3perst/1 -> boost_pressure_map/1(fuel_rate_mm3perst)
  boost_pressure_map/1(intake_manifold_pressure) -> intake_manifold_pressure_ref/1

== system KD_cl_harness_forthao/pre-throttle manifold/p_preThrottle/Cus_integrator ==
  in : Inport
  p_prethrottle (kPa)1 : Integrator  InitialCondition=IV.p_prethrottle  UpperSaturationLimit=maxL.p_PreThrottle  LowerSaturationLimit=minL.p_PreThrottle
  p_preThrottle : Outport
  wires:
  p_prethrottle (kPa)1/1 -> p_preThrottle/1
  in/1 -> p_prethrottle (kPa)1/1

== system KD_cl_harness_forthao/EGR Throttle/EGR Throttle/Throttle Model2/Air Model_map_use ==
  TA[deg] : Inport
  Ne[rpm] : Inport  Port=2
  Pim[Pa] : Inport  Port=3
  Tim[K] : Inport  Port=4
  Pa[Pa] : Inport  Port=5
  Ta[K] : Inport  Port=6
  R_im : Inport  Port=7
  R_a : Inport  Port=8
  Back-Flow : Subsystem
  Forward-Flow : Subsystem
  Gain : Gain  Gain=-1
  Product : Product  Inputs=/*  SaturateOnIntegerOverflow=on  RndMeth=Zero  InputSameDT=on  OutDataTypeStr=Inherit: Same as first input
  Product1 : Product  Inputs=*//  SaturateOnIntegerOverflow=on  RndMeth=Zero  InputSameDT=on  OutDataTypeStr=Inherit: Same as first input
  Product3 : Product  Inputs=*//  SaturateOnIntegerOverflow=on  RndMeth=Zero  InputSameDT=on  OutDataTypeStr=Inherit: Same as first input
  Switch : Switch  Threshold=1  SaturateOnIntegerOverflow=on  InputSameDT=on
  mt[kg/sec] : Outport
  forwardmt : Outport  Port=2
  backwardmt : Outport  Port=3
  wires:
  Product1/1 -> Forward-Flow/1(Ro_a)
  Switch/1 -> mt[kg/sec]/1
  Product/1 -> Switch/2
  TA[deg]/1 -> Forward-Flow/2(TA[deg]), Back-Flow/1(TA[deg])
  [Pa] -> Product/2, Forward-Flow/4(Pa), Back-Flow/4(Pa)
  Pim[Pa]/1 -> Forward-Flow/5(Pm), Product/1, Back-Flow/5(Pm), Product3/1
  Pa[Pa]/1 -> [Pa]
  Ta[K]/1 -> [Ta]
  R_a/1 -> [Ra]
  R_im/1 -> [Rim]
  [Ra] -> Product1/3
  [Pa] -> Product1/1
  [Ta] -> Product1/2
  [Rim] -> Product3/3
  Tim[K]/1 -> Product3/2
  Forward-Flow/1(mt_dot[kg/s]) -> Switch/1, forwardmt/1
  Product3/1 -> Back-Flow/3(Ro_m)
  Back-Flow/1(mt_dot[kg/s]) -> Gain/1
  Ne[rpm]/1 -> Forward-Flow/3(Ne[rpm]), Back-Flow/2(Ne[rpm])
  Gain/1 -> Switch/3, backwardmt/1

== system KD_cl_harness_forthao/EGR Valve/SVR EGR/EGR_model/Air Model_map_use ==
  TA[deg] : Inport
  Ne[rpm] : Inport  Port=2
  Pim[Pa] : Inport  Port=3
  Tim[K] : Inport  Port=4
  Pa[Pa] : Inport  Port=5
  Ta[K] : Inport  Port=6
  R_im : Inport  Port=7
  R_a : Inport  Port=8
  Back-Flow : Subsystem
  Forward-Flow : Subsystem
  Gain : Gain  Gain=-1
  Product : Product  Inputs=/*  SaturateOnIntegerOverflow=on  RndMeth=Zero  InputSameDT=on  OutDataTypeStr=Inherit: Same as first input
  Product1 : Product  Inputs=*//  SaturateOnIntegerOverflow=on  RndMeth=Zero  InputSameDT=on  OutDataTypeStr=Inherit: Same as first input
  Product3 : Product  Inputs=*//  SaturateOnIntegerOverflow=on  RndMeth=Zero  InputSameDT=on  OutDataTypeStr=Inherit: Same as first input
  Switch : Switch  Threshold=1  SaturateOnIntegerOverflow=on  InputSameDT=on
  mt[kg/sec] : Outport
  forwardmt : Outport  Port=2
  wires:
  Ne[rpm]/1 -> Back-Flow/2(Ne[rpm]), Forward-Flow/3(Ne[rpm])
  Back-Flow/1(mt_dot[kg/s]) -> Gain/1  "rv"
  Product3/1 -> Back-Flow/3(Ro_m)
  Forward-Flow/1(mt_dot[kg/s]) -> forwardmt/1, Switch/1  "ff"
  Tim[K]/1 -> Product3/2
  [Rim] -> Product3/3
  [Ta] -> Product1/2
  [Pa] -> Product1/1
  [Ra] -> Product1/3
  R_im/1 -> [Rim]
  R_a/1 -> [Ra]
  Ta[K]/1 -> [Ta]
  Pa[Pa]/1 -> [Pa]
  Pim[Pa]/1 -> Product3/1, Back-Flow/5(Pm), Product/1, Forward-Flow/5(Pm)
  [Pa] -> Back-Flow/4(Pa), Forward-Flow/4(Pa), Product/2
  TA[deg]/1 -> Back-Flow/1(TA[deg]), Forward-Flow/2(TA[deg])
  Product/1 -> Switch/2  "pr_exhaust_by_intake"
  Switch/1 -> mt[kg/sec]/1
  Product1/1 -> Forward-Flow/1(Ro_a)
  Gain/1 -> Switch/3
